simulink model "Hurwitzovo_kriterium_stability"  (R2022b)
settings: Solver=VariableStepAuto  StartTime=0.0  StopTime=25.0  MaxStep=0.01  MinStep=0.001  RelTol=1e-3
settings Model: Creator=honza  LastModifiedBy=honza
settings SolverCC: InitialStep=0.01

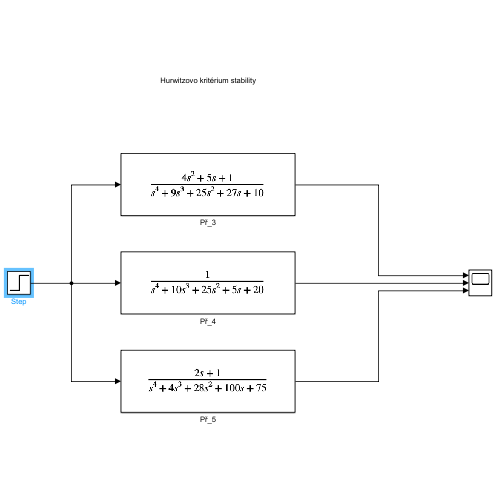
[thumbnail: Simulink's stored preview of the top-level diagram]
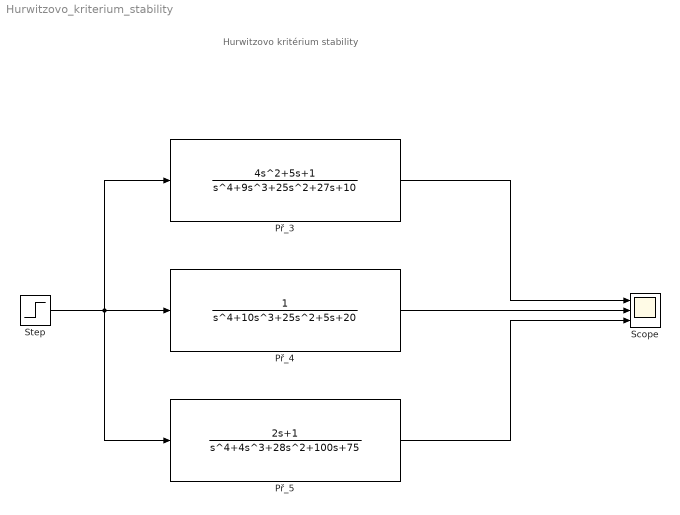
== system Hurwitzovo_kriterium_stability ==
  note: Hurwitzovo kritérium stability
  Př_3 : TransferFcn  Numerator=[4 5 1]  Denominator=[1 9 25 27 10]
  Př_4 : TransferFcn  Denominator=[1 10 25 5 20]
  Př_5 : TransferFcn  Numerator=[2 1]  Denominator=[1 4 28 100 75]
  Scope : Scope  NumInputPorts=3
  Step : Step  Time=0  SampleTime=0
  wires:
  Step/1 -> Př_5/1, Př_3/1, Př_4/1
  Př_3/1 -> Scope/1
  Př_4/1 -> Scope/2
  Př_5/1 -> Scope/3
